simulink model "p9"  (R2017b)
settings: Solver=VariableStepAuto  StartTime=0.0  StopTime=10.0  RelTol=1e-3
values from neighbouring files (symbols this model uses):
  dq = [dq1;dq2]    [dJ_dq_symb.m]    (also in derivative_position.m; initial_values.m; robot.m; tau_c.m = [entradas(9); entradas(10)])
settings Model: Creator=Rita Monteiro  LastModifiedBy=Rita Monteiro
settings DataIOCC: SaveFormat=Array

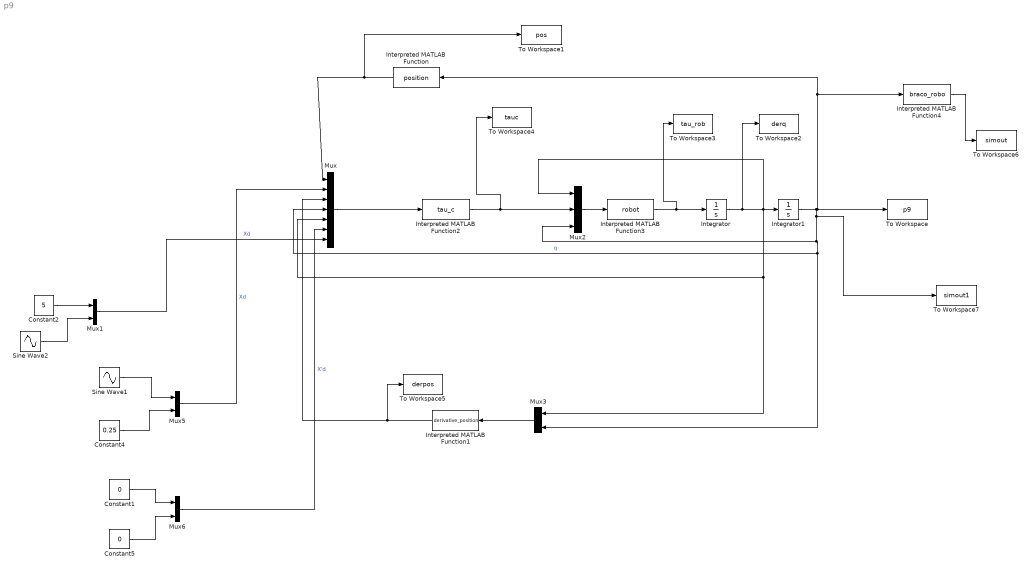
== system p9 ==
  Constant1 : Constant  Value=0
  Constant2 : Constant  Value=5
  Constant4 : Constant  Value=0.25
  Constant5 : Constant  Value=0
  Integrator : Integrator  InitialCondition=dq  IgnoreLimit=on
  Integrator1 : Integrator  InitialCondition=[pi/2;-pi/4]
  Interpreted MATLAB Function : MATLABFcn  MATLABFcn=position
  Interpreted MATLAB Function1 : MATLABFcn  MATLABFcn=derivative_position
  Interpreted MATLAB Function2 : MATLABFcn  MATLABFcn=tau_c
  Interpreted MATLAB Function3 : MATLABFcn  MATLABFcn=robot
  Interpreted MATLAB Function4 : MATLABFcn  MATLABFcn=braco_robo  OutputDimensions=1
  Mux : Mux  Inputs=7
  Mux{1,3,5..6} (4 alike) : Mux  Inputs=2
  Mux2 : Mux  Inputs=3
  Sine Wave1 : Sin  Amplitude=0.3  Bias=0.05  Frequency=pi/4  Phase=pi/2  SampleTime=0
  Sine Wave2 : Sin  Frequency=2*pi  Phase=pi/2  SampleTime=0
  To Workspace : ToWorkspace  VariableName=p9  SaveFormat=Structure With Time  SampleTime=-1
  To Workspace1 : ToWorkspace  VariableName=pos  SaveFormat=Timeseries  SampleTime=-1
  To Workspace2 : ToWorkspace  VariableName=derq  SaveFormat=Timeseries  SampleTime=-1
  To Workspace3 : ToWorkspace  VariableName=tau_rob  SaveFormat=Timeseries  SampleTime=-1
  To Workspace4 : ToWorkspace  VariableName=tauc  SaveFormat=Timeseries  SampleTime=-1
  To Workspace5 : ToWorkspace  VariableName=derpos  SaveFormat=Timeseries  SampleTime=-1
  To Workspace6 : ToWorkspace  VariableName=simout  SaveFormat=Timeseries  SampleTime=-1
  To Workspace7 : ToWorkspace  VariableName=simout1  SaveFormat=Timeseries  SampleTime=-1
  wires:
  Interpreted MATLAB Function/1 -> To Workspace1/1, Mux/1
  Mux/1 -> Interpreted MATLAB Function2/1
  Mux2/1 -> Interpreted MATLAB Function3/1
  Mux3/1 -> Interpreted MATLAB Function1/1
  Interpreted MATLAB Function2/1 -> To Workspace4/1, Mux2/2
  Interpreted MATLAB Function3/1 -> To Workspace3/1, Integrator/1
  Integrator/1 -> To Workspace2/1, Integrator1/1, Mux/5, Mux3/1, Mux2/1
  Integrator1/1 -> To Workspace/1, Interpreted MATLAB Function/1, Interpreted MATLAB Function4/1, To Workspace7/1, Mux/4, Mux3/2, Mux2/3  "q"
  Interpreted MATLAB Function1/1 -> To Workspace5/1, Mux/3
  Mux6/1 -> Mux/6  "X'd"
  Mux5/1 -> Mux/2  "Xd"
  Constant5/1 -> Mux6/2
  Constant4/1 -> Mux5/2
  Sine Wave1/1 -> Mux5/1
  Constant1/1 -> Mux6/1
  Interpreted MATLAB Function4/1 -> To Workspace6/1
  Constant2/1 -> Mux1/1
  Sine Wave2/1 -> Mux1/2
  Mux1/1 -> Mux/7  "Xd"
